simulink model "Tests"  (R2017b)
settings: Solver=FixedStepDiscrete  StartTime=0.0  StopTime=time  FixedStep=0.0025  RelTol=1e-3
InitFcn:
  | time = Data(size(Data,1),1);
values from neighbouring files (symbols this model uses):
  Data = [0 0.0025 0.005 0.0075 0.01 0.0125 0.015 0.0175 0.02 0.0225 0.025 0.0275 ... (231351 elements, 3453x67)]    [apAerobi_0.mat]    (also in apAerobi_3.mat = [0 0.0025 0.005 0.0075 0.01 0.0125 0.015 0.0175 0.02 0.0225 ; apAerobi_4.mat = [0 0.0025 0.005 0.0075 0.01 0.0125 0.015 0.0175 0.02 0.0225 )
libraries: simulink x25
settings Model: Creator=GRVC  LastModifiedBy=root
settings CodeAppCC: StateflowObjectComments=on

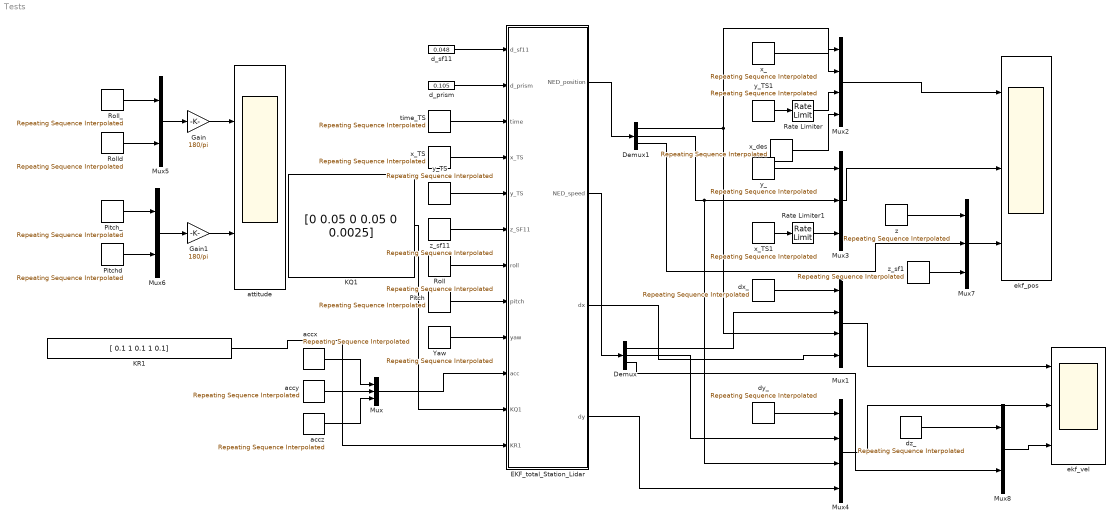
== system Tests ==
  Demux : Demux  Outputs=3
  Demux1 : Demux  Outputs=3
  EKF_total_Station_Lidar : Subsystem
  Gain : Gain  Gain=180/pi
  Gain1 : Gain  Gain=180/pi
  KQ1 : Constant  Value="[0 0.05  0 0.05 0 0.0025]"
  KR1 : Constant  Value=[ 0.1 1 0.1 1 0.1]
  Mux : Mux  Inputs=3
  Mux1 : Mux
  Mux2 : Mux
  Mux3 : Mux  Inputs=3
  Mux4 : Mux
  Mux5 : Mux  Inputs=2
  Mux6 : Mux  Inputs=2
  Mux7 : Mux  Inputs=3
  Mux8 : Mux  Inputs=2
  Pitch : simulink/Sources/Repeating Sequence Interpolated  OutValues=Data(:,3)  TimeValues=Data(:,1)  LookUpMeth=Interpolation-Use End Values  tsamp=0.0025  OutMin=[]  OutMax=[]  OutDataTypeStr=double  OutputDataTypeScalingMode=double  OutDataType=fixdt(0,8)  OutScaling=2^-10
  Pitch_ : simulink/Sources/Repeating Sequence Interpolated  OutValues=Data(:,3)  TimeValues=Data(:,1)  LookUpMeth=Interpolation-Use End Values  tsamp=0.0025  OutMin=[]  OutMax=[]  OutDataTypeStr=double  OutputDataTypeScalingMode=double  OutDataType=fixdt(0,8)  OutScaling=2^-10
  Pitchd : simulink/Sources/Repeating Sequence Interpolated  OutValues=Data(:,49)  TimeValues=Data(:,1)  LookUpMeth=Interpolation-Use End Values  tsamp=0.0025  OutMin=[]  OutMax=[]  OutDataTypeStr=double  OutputDataTypeScalingMode=double  OutDataType=fixdt(0,8)  OutScaling=2^-10
  Rate Limiter : RateLimiter  RisingSlewLimit=10  FallingSlewLimit=-10  SampleTimeMode=inherited
  Rate Limiter1 : RateLimiter  RisingSlewLimit=10  FallingSlewLimit=-10  SampleTimeMode=inherited
  Roll : simulink/Sources/Repeating Sequence Interpolated  OutValues=Data(:,2)  TimeValues=Data(:,1)  LookUpMeth=Interpolation-Use End Values  tsamp=0.0025  OutMin=[]  OutMax=[]  OutDataTypeStr=double  OutputDataTypeScalingMode=double  OutDataType=fixdt(0,8)  OutScaling=2^-10
  Roll_ : simulink/Sources/Repeating Sequence Interpolated  OutValues=Data(:,2)  TimeValues=Data(:,1)  LookUpMeth=Interpolation-Use End Values  tsamp=0.0025  OutMin=[]  OutMax=[]  OutDataTypeStr=double  OutputDataTypeScalingMode=double  OutDataType=fixdt(0,8)  OutScaling=2^-10
  Rolld : simulink/Sources/Repeating Sequence Interpolated  OutValues=Data(:,48)  TimeValues=Data(:,1)  LookUpMeth=Interpolation-Use End Values  tsamp=0.0025  OutMin=[]  OutMax=[]  OutDataTypeStr=double  OutputDataTypeScalingMode=double  OutDataType=fixdt(0,8)  OutScaling=2^-10
  Yaw : simulink/Sources/Repeating Sequence Interpolated  OutValues=Data(:,4)  TimeValues=Data(:,1)  LookUpMeth=Interpolation-Use End Values  tsamp=0.0025  OutMin=[]  OutMax=[]  OutDataTypeStr=double  OutputDataTypeScalingMode=double  OutDataType=fixdt(0,8)  OutScaling=2^-10
  accx : simulink/Sources/Repeating Sequence Interpolated  OutValues=Data(:,8)  TimeValues=Data(:,1)  LookUpMeth=Interpolation-Use End Values  tsamp=0.0025  OutMin=[]  OutMax=[]  OutDataTypeStr=double  OutputDataTypeScalingMode=double  OutDataType=fixdt(0,8)  OutScaling=2^-10
  accy : simulink/Sources/Repeating Sequence Interpolated  OutValues=Data(:,9)  TimeValues=Data(:,1)  LookUpMeth=Interpolation-Use End Values  tsamp=0.0025  OutMin=[]  OutMax=[]  OutDataTypeStr=double  OutputDataTypeScalingMode=double  OutDataType=fixdt(0,8)  OutScaling=2^-10
  accz : simulink/Sources/Repeating Sequence Interpolated  OutValues=Data(:,10)  TimeValues=Data(:,1)  LookUpMeth=Interpolation-Use End Values  tsamp=0.0025  OutMin=[]  OutMax=[]  OutDataTypeStr=double  OutputDataTypeScalingMode=double  OutDataType=fixdt(0,8)  OutScaling=2^-10
  attitude : Scope  NumInputPorts=2
  d_prism : Constant  Value=0.105
  d_sf11 : Constant  Value=0.048
  dx_ : simulink/Sources/Repeating Sequence Interpolated  OutValues=Data(:,33)  TimeValues=Data(:,1)  LookUpMeth=Interpolation-Use End Values  tsamp=0.0025  OutMin=[]  OutMax=[]  OutDataTypeStr=double  OutputDataTypeScalingMode=double  OutDataType=fixdt(0,8)  OutScaling=2^-10
  dy_ : simulink/Sources/Repeating Sequence Interpolated  OutValues=Data(:,34)  TimeValues=Data(:,1)  LookUpMeth=Interpolation-Use End Values  tsamp=0.0025  OutMin=[]  OutMax=[]  OutDataTypeStr=double  OutputDataTypeScalingMode=double  OutDataType=fixdt(0,8)  OutScaling=2^-10
  dz_ : simulink/Sources/Repeating Sequence Interpolated  OutValues=Data(:,35)  TimeValues=Data(:,1)  LookUpMeth=Interpolation-Use End Values  tsamp=0.0025  OutMin=[]  OutMax=[]  OutDataTypeStr=double  OutputDataTypeScalingMode=double  OutDataType=fixdt(0,8)  OutScaling=2^-10
  ekf_pos : Scope  NumInputPorts=3
  ekf_vel : Scope  NumInputPorts=3
  time_TS : simulink/Sources/Repeating Sequence Interpolated  OutValues=Data(:,40)  TimeValues=Data(:,1)  LookUpMeth=Interpolation-Use End Values  tsamp=0.0025  OutMin=[]  OutMax=[]  OutDataTypeStr=double  OutputDataTypeScalingMode=double  OutDataType=fixdt(0,8)  OutScaling=2^-10
  x_ : simulink/Sources/Repeating Sequence Interpolated  OutValues=Data(:,30)  TimeValues=Data(:,1)  LookUpMeth=Interpolation-Use End Values  tsamp=0.0025  OutMin=[]  OutMax=[]  OutDataTypeStr=double  OutputDataTypeScalingMode=double  OutDataType=fixdt(0,8)  OutScaling=2^-10
  x_TS : simulink/Sources/Repeating Sequence Interpolated  OutValues=Data(:,37)  TimeValues=Data(:,1)  LookUpMeth=Interpolation-Use End Values  tsamp=0.0025  OutMin=[]  OutMax=[]  OutDataTypeStr=double  OutputDataTypeScalingMode=double  OutDataType=fixdt(0,8)  OutScaling=2^-10
  x_TS1 : simulink/Sources/Repeating Sequence Interpolated  OutValues=Data(:,37)  TimeValues=Data(:,1)  LookUpMeth=Interpolation-Use End Values  tsamp=0.0025  OutMin=[]  OutMax=[]  OutDataTypeStr=double  OutputDataTypeScalingMode=double  OutDataType=fixdt(0,8)  OutScaling=2^-10
  x_des : simulink/Sources/Repeating Sequence Interpolated  OutValues=Data(:,41)  TimeValues=Data(:,1)  LookUpMeth=Interpolation-Use End Values  tsamp=0.0025  OutMin=[]  OutMax=[]  OutDataTypeStr=double  OutputDataTypeScalingMode=double  OutDataType=fixdt(0,8)  OutScaling=2^-10
  y_ : simulink/Sources/Repeating Sequence Interpolated  OutValues=Data(:,31)  TimeValues=Data(:,1)  LookUpMeth=Interpolation-Use End Values  tsamp=0.0025  OutMin=[]  OutMax=[]  OutDataTypeStr=double  OutputDataTypeScalingMode=double  OutDataType=fixdt(0,8)  OutScaling=2^-10
  y_TS : simulink/Sources/Repeating Sequence Interpolated  OutValues=Data(:,38)  TimeValues=Data(:,1)  LookUpMeth=Interpolation-Use End Values  tsamp=0.0025  OutMin=[]  OutMax=[]  OutDataTypeStr=double  OutputDataTypeScalingMode=double  OutDataType=fixdt(0,8)  OutScaling=2^-10
  y_TS1 : simulink/Sources/Repeating Sequence Interpolated  OutValues=Data(:,38)  TimeValues=Data(:,1)  LookUpMeth=Interpolation-Use End Values  tsamp=0.0025  OutMin=[]  OutMax=[]  OutDataTypeStr=double  OutputDataTypeScalingMode=double  OutDataType=fixdt(0,8)  OutScaling=2^-10
  z : simulink/Sources/Repeating Sequence Interpolated  OutValues=Data(:,32)  TimeValues=Data(:,1)  LookUpMeth=Interpolation-Use End Values  tsamp=0.0025  OutMin=[]  OutMax=[]  OutDataTypeStr=double  OutputDataTypeScalingMode=double  OutDataType=fixdt(0,8)  OutScaling=2^-10
  z_sf1 : simulink/Sources/Repeating Sequence Interpolated  OutValues=Data(:,36)  TimeValues=Data(:,1)  LookUpMeth=Interpolation-Use End Values  tsamp=0.0025  OutMin=[]  OutMax=[]  OutDataTypeStr=double  OutputDataTypeScalingMode=double  OutDataType=fixdt(0,8)  OutScaling=2^-10
  z_sf11 : simulink/Sources/Repeating Sequence Interpolated  OutValues=Data(:,36)  TimeValues=Data(:,1)  LookUpMeth=Interpolation-Use End Values  tsamp=0.0025  OutMin=[]  OutMax=[]  OutDataTypeStr=double  OutputDataTypeScalingMode=double  OutDataType=fixdt(0,8)  OutScaling=2^-10
  wires:
  accy/1 -> Mux/2
  accz/1 -> Mux/3
  accx/1 -> Mux/1
  Mux/1 -> EKF_total_Station_Lidar/10(acc)
  time_TS/1 -> EKF_total_Station_Lidar/3(time)
  d_sf11/1 -> EKF_total_Station_Lidar/1(d_sf11)
  d_prism/1 -> EKF_total_Station_Lidar/2(d_prism)
  z_sf11/1 -> EKF_total_Station_Lidar/6(z_SF11)
  Roll/1 -> EKF_total_Station_Lidar/7(roll)
  Pitch/1 -> EKF_total_Station_Lidar/8(pitch)
  Yaw/1 -> EKF_total_Station_Lidar/9(yaw)
  Mux2/1 -> ekf_pos/1
  Mux3/1 -> ekf_pos/2
  Mux1/1 -> ekf_vel/1
  Mux4/1 -> ekf_vel/2
  dx_/1 -> Mux1/1
  EKF_total_Station_Lidar/1(NED_position) -> Demux1/1
  Demux/1 -> Mux1/2
  Demux/2 -> Mux4/2
  x_/1 -> Mux2/1
  y_/1 -> Mux3/1
  Demux/3 -> Mux8/2
  Demux1/3 -> Mux7/2
  dy_/1 -> Mux4/1
  y_TS1/1 -> Rate Limiter/1
  x_TS1/1 -> Rate Limiter1/1
  Rate Limiter/1 -> Mux2/3
  Rate Limiter1/1 -> Mux3/3
  Rolld/1 -> Mux5/2
  Roll_/1 -> Mux5/1
  Mux5/1 -> Gain/1
  Mux6/1 -> Gain1/1
  Pitchd/1 -> Mux6/2
  Pitch_/1 -> Mux6/1
  Demux1/1 -> Mux1/3, Mux2/2
  Demux1/2 -> Mux4/3, Mux3/2
  y_TS/1 -> EKF_total_Station_Lidar/5(y_TS)
  x_TS/1 -> EKF_total_Station_Lidar/4(x_TS)
  EKF_total_Station_Lidar/2(NED_speed) -> Demux/1
  KR1/1 -> EKF_total_Station_Lidar/12(KR1)
  KQ1/1 -> EKF_total_Station_Lidar/11(KQ1)
  Mux7/1 -> ekf_pos/3
  z_sf1/1 -> Mux7/3
  z/1 -> Mux7/1
  Mux8/1 -> ekf_vel/3
  dz_/1 -> Mux8/1
  Gain/1 -> attitude/1
  Gain1/1 -> attitude/2
  x_des/1 -> Mux2/4
  EKF_total_Station_Lidar/3(dx) -> Mux1/4
  EKF_total_Station_Lidar/4(dy) -> Mux4/4

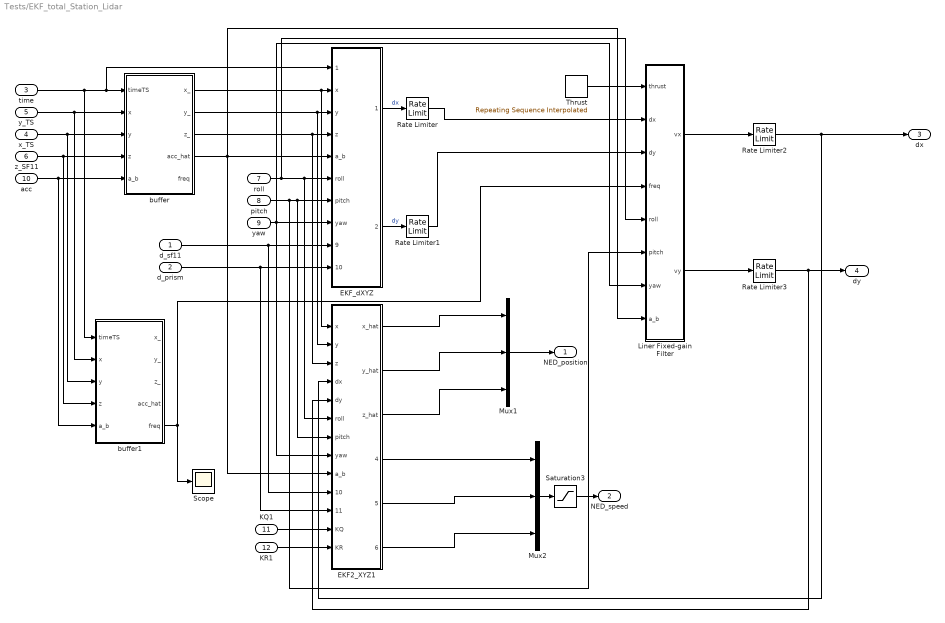
== system Tests/EKF_total_Station_Lidar ==
  d_sf11 : Inport
  d_prism : Inport  Port=2
  time : Inport  Port=3
  x_TS : Inport  Port=4
  y_TS : Inport  Port=5
  z_SF11 : Inport  Port=6
  roll : Inport  Port=7
  pitch : Inport  Port=8
  yaw : Inport  Port=9
  acc : Inport  Port=10
  KQ1 : Inport  Port=11
  KR1 : Inport  Port=12
  EKF2_XYZ1 : MATLAB Function  TreatAsAtomicUnit=on
  EKF_dXYZ : MATLAB Function  TreatAsAtomicUnit=on
  Liner Fixed-gain Filter : MATLAB Function  TreatAsAtomicUnit=on
  Mux1 : Mux  Inputs=3
  Mux2 : Mux  Inputs=3
  Rate Limiter{,1..3} (4 alike) : RateLimiter  RisingSlewLimit=5  FallingSlewLimit=-5  SampleTimeMode=inherited
  Saturation3 : Saturate  UpperLimit=10  LowerLimit=-10
  Scope : Scope
  Thrust : simulink/Sources/Repeating Sequence Interpolated  OutValues=Data(:,45)  TimeValues=Data(:,1)  LookUpMeth=Interpolation-Use End Values  tsamp=0.0025  OutMin=[]  OutMax=[]  OutDataTypeStr=double  OutputDataTypeScalingMode=double  OutDataType=fixdt(0,8)  OutScaling=2^-10
  buffer : MATLAB Function  TreatAsAtomicUnit=on
  buffer1 : MATLAB Function  TreatAsAtomicUnit=on
  NED_position : Outport
  NED_speed : Outport  Port=2
  dx : Outport  Port=3
  dy : Outport  Port=4
  wires:
  Mux1/1 -> NED_position/1
  Mux2/1 -> Saturation3/1
  x_TS/1 -> buffer1/3(y), buffer/3(y)
  y_TS/1 -> buffer/2(x), buffer1/2(x)
  z_SF11/1 -> buffer1/4(z), buffer/4(z)
  acc/1 -> buffer1/5(a_b), buffer/5(a_b)
  buffer/4(acc_hat) -> EKF2_XYZ1/9(a_b), Liner Fixed-gain Filter/8(a_b), EKF_dXYZ/5(a_b)
  EKF_dXYZ/1(dx_hat) -> Rate Limiter/1  "dx"
  EKF_dXYZ/2(dy_hat) -> Rate Limiter1/1  "dy"
  roll/1 -> Liner Fixed-gain Filter/5(roll), EKF2_XYZ1/6(roll), EKF_dXYZ/6(roll)
  pitch/1 -> Liner Fixed-gain Filter/6(pitch), EKF2_XYZ1/7(pitch), EKF_dXYZ/7(pitch)
  yaw/1 -> EKF2_XYZ1/8(yaw), Liner Fixed-gain Filter/7(yaw), EKF_dXYZ/8(yaw)
  d_sf11/1 -> EKF2_XYZ1/10(d_sf11), EKF_dXYZ/9(d_sf11)
  d_prism/1 -> EKF2_XYZ1/11(d_prism), EKF_dXYZ/10(d_prism)
  KQ1/1 -> EKF2_XYZ1/12(KQ)
  KR1/1 -> EKF2_XYZ1/13(KR)
  EKF2_XYZ1/1(x_hat) -> Mux1/1
  EKF2_XYZ1/2(y_hat) -> Mux1/2
  EKF2_XYZ1/3(z_hat) -> Mux1/3
  EKF2_XYZ1/4(dx_hat) -> Mux2/1
  EKF2_XYZ1/5(dy_hat) -> Mux2/2
  EKF2_XYZ1/6(dz_hat) -> Mux2/3
  Saturation3/1 -> NED_speed/1
  time/1 -> buffer1/1(timeTS), EKF_dXYZ/1(timeTS), buffer/1(timeTS)
  buffer/2(y_) -> EKF2_XYZ1/2(y), EKF_dXYZ/3(y)
  buffer/1(x_) -> EKF2_XYZ1/1(x), EKF_dXYZ/2(x)
  buffer/3(z_) -> EKF2_XYZ1/3(z), EKF_dXYZ/4(z)
  Liner Fixed-gain Filter/1(vx) -> Rate Limiter2/1
  Liner Fixed-gain Filter/2(vy) -> Rate Limiter3/1
  Rate Limiter/1 -> Liner Fixed-gain Filter/2(dx)
  Rate Limiter1/1 -> Liner Fixed-gain Filter/3(dy)
  Thrust/1 -> Liner Fixed-gain Filter/1(thrust)
  Rate Limiter2/1 -> EKF2_XYZ1/4(dx), dx/1
  Rate Limiter3/1 -> EKF2_XYZ1/5(dy), dy/1
  buffer1/5(freq) -> Liner Fixed-gain Filter/4(freq), Scope/1

== matlab function Tests/EKF_total_Station_Lidar/EKF_dXYZ ==
  data: timeTS input; x input; y input; z input; a_b input; roll input; pitch input; yaw input; d_sf11 input; d_prism input; dx_hat output; dy_hat output
function [dx_hat,dy_hat] = EKF(timeTS,x,y,z,a_b,roll,pitch,yaw,d_sf11,d_prism)

dt = 0.0025;


a_I = [(a_b(2)-sin(pitch))*cos(yaw)-sin(yaw)*((a_b(1)+sin(roll)*cos(pitch)));
        sin(yaw)*(a_b(2)-sin(pitch))+cos(yaw)*((a_b(1)+sin(roll)*cos(pitch)));
        a_b(3)-cos(roll)*cos(pitch)];

persistent time timeTS0 dx_k dP_k queue_dx queue_dP index Ndata timefreq
if isempty(dx_k) || isempty(dP_k)||isempty(time)|| isempty(timeTS0)|| isempty(queue_dx)|| isempty(queue_dP)|| isempty(index)|| isempty(timefreq)|| isempty(Ndata)

    dx_k = [0;0;0;0;z;0];  
    dP_k = eye(6,6);
    queue_dx = zeros(6,10);
    queue_dP = zeros(6,6,10);

    time = 0;
    timeTS0 = timeTS;
    index = 0;
    timefreq = 0;
    Ndata = 0;

else
    z_corr = d_sf11*sin(roll);
    x_corr = d_prism*cos(yaw);
    y_corr = d_prism*sin(yaw);
    z = (z*cos(roll)+z_corr)*cos(pitch);
    x = x+x_corr;
    y = y+y_corr;
    if timeTS~=0
        if timeTS0~=timeTS
            T = time;
            time = 0;
            timeTS0=timeTS;

            dF = [1 T  0 0  0 0;
                  0 1  0 0  0 0;
                  0 0  1 T  0 0;
                  0 0  0 1  0 0;
                  0 0  0 0  1 T;
                  0 0  0 0  0 1];
            dB = [0.5*T^2       0       0;
                       T       0       0;
                       0  0.5*T^2       0;
                       0        T       0;
                       0        0 0.5*T^2;
                       0        0       T];
            dw_k = [a_I(1);a_I(2);a_I(3)];
            dz_k = [x;y;z];
            dy_k = [dx_k(1);dx_k(3);dx_k(5)];
            dH =[1   0 0  0 0  0;
                0   0 1  0 0  0;
                0   0 0  0 1  0];
            dQ = diag([0 0.05  0 0.05 0 0.05]);
            dR = diag([0.001 0.001 0.001]);
            
        %---------PREDICTION---------%
        %1. Project the state ahead
            dx_k = dF * dx_k + dB * dw_k;
        %2. Project the error covariance ahead
            dP_k = dF * dP_k * dF' + dQ;  
        %--------CORRECTION----------%
        %1. Compute the Kalman Gain
            dK_k = dP_k * dH' / (dH*dP_k*dH' + dR);
            %resid = [sqrt(x0^2+y0^2);atan2(y0,x0);z0] - y_k;
            dresid = dz_k - dy_k;
        %2. Update the estimate via measurement
            dx_k = dx_k +dK_k * dresid;
        %3. Update the error covariance
            dP_k = (eye(size(dK_k,1)) - dK_k * dH) * dP_k;
            
            index = index + 1;

            if index > 10
                queue_dx(:,1) =  dx_k;
                queue_dP(:,:,1) = dP_k;
                index = 1;
            else
                queue_dx(:,index) =  dx_k;
                queue_dP(:,:,index) = dP_k;
            end

        else
            time = time + dt;
        end
   end  

end
dx_hat = dx_k(2);
dy_hat = dx_k(4);

== matlab function Tests/EKF_total_Station_Lidar/buffer1 ==
  data: timeTS input; x_ output; x input; y input; z input; y_ output; z_ output; acc_hat output; freq output; a_b input
function [x_,y_,z_,acc_hat,freq] = data_buffer(timeTS,x,y,z,a_b)

dt = 0.0025;
persistent buffer time index counter t0 total acc_
if isempty(buffer)||isempty(time)||isempty(index)||isempty(counter)||isempty(t0)||isempty(total)||isempty(acc_)
    buffer = zeros(3,20);
    
    time = 0;
    index = 1;
    counter = zeros(1,20);
    if timeTS ~= 0
        buffer(:,index) = [x;y;z];
        counter(1) = 1;
    end
    total = 0;
    t0 = timeTS;
   
    acc_ = [0;0;1];
        
else
    alpha = 0.2;
    a_b = a_b/norm(a_b);
    acc_ = (a_b * alpha) + (acc_ * (1.0 - alpha));
    time = time + dt;
    if time > 0.05
        time = 0;
        if (buffer(1,index) ~= x || buffer(2,index) ~= y )
            buffer(:,index) = [x;y;z];
            counter(index) = 1;
        else

            buffer(:,index) = [x;y;z];
            counter(index) = 0;
        end
        if index == 20
            index = 1;
        else
            index = index + 1;
        end

    end
 
    
end
    freq =sum(counter);
    if freq > 20
        freq = 20;
    end
    if isnan(x) || isnan(y) || isinf(x) || isinf(y) || abs(x) > 50 || abs(y) > 50
        if index <= 1
            x_ = buffer(1,10);
            y_ = buffer(2,10);
        else       
            x_ = buffer(1,index-1);
            y_ = buffer(2,index-1);
        end
        z_ = z;
    else
        if z < 0.3
            z_ = 0.3;
        else
            z_ = z;
        end
        x_ = x;
        y_ = y;   
    end
    acc_hat = acc_;
end

== matlab function Tests/EKF_total_Station_Lidar/buffer ==
  data: timeTS input; x_ output; x input; y input; z input; y_ output; z_ output; acc_hat output; freq output; a_b input
function [x_,y_,z_,acc_hat,freq] = data_buffer(timeTS,x,y,z,a_b)

dt = 0.0025;
persistent buffer time index counter t0 total acc_
if isempty(buffer)||isempty(time)||isempty(index)||isempty(counter)||isempty(t0)||isempty(total)||isempty(acc_)
    buffer = zeros(3,20);
    time = 0;
    index = 1;
    counter = 0;
    if timeTS ~= 0
        buffer(:,index) = [x;y;z];
        counter = 1;
    end
    total = counter;
    t0 = timeTS;
   
    acc_ = [0;0;1];
        
else
    alpha = 0.2;
    a_b = a_b/norm(a_b);
    acc_ = (a_b * alpha) + (acc_ * (1.0 - alpha));
    time = time + dt;
    if timeTS ~= 0 && timeTS <= 1e13        
        if time > 0.5
            %counter = index - 1;
            total = counter;
            counter = 0;
            time = 0;                  
            index = 0;
        else
            
            if index == 0
                if (buffer(1,10) ~= x || buffer(2,10) ~= y )
                    counter = counter+1;
                    buffer(:,1) = [x;y;z];
                    index = 1;
                end
            elseif index >= 10  
                if (buffer(1,10) ~= x || buffer(2,10) ~= y )
                    counter = counter+1;
                    buffer(:,1) = [x;y;z];
                    index = 1;
                end
            else
                if (buffer(1,index) ~= x || buffer(2,index) ~= y )
                    index = index + 1;
                    counter = counter+1;                   
                    buffer(:,index) = [x;y;z];                    
                end
            end
        end

    elseif timeTS == 0
        if time > 0.5
            time = 0;
            index = 0;
            total = counter;
            counter = 0;
        end
    else
        if time > 0.5
            %counter = index - 1;
            total = counter;
            counter = 0;
            time = 0;
            index = 0;
        end
        
    end

    
end
    freq =total/0.5;
    if freq > 20
        freq = 20;
    end
    if isnan(x) || isnan(y) || isinf(x) || isinf(y) || abs(x) > 50 || abs(y) > 50
        if index <= 1
            x_ = buffer(1,10);
            y_ = buffer(2,10);
        else       
            x_ = buffer(1,index-1);
            y_ = buffer(2,index-1);
        end
        z_ = z;
    else
        if z < 0.3
            z_ = 0.3;
        else
            z_ = z;
        end
        x_ = x;
        y_ = y;   
    end
    acc_hat = acc_;
end

== matlab function Tests/EKF_total_Station_Lidar/Liner Fixed-gain Filter ==
  data: thrust input; dx input; dy input; freq input; roll input; pitch input; yaw input; a_b input; vx output; vy output
function [vx,vy] = linear_Fixed_Gain_Filter(thrust,dx,dy,freq,roll,pitch,yaw,a_b)

dt = 0.0025;
m = 2.5;
mu = 0.87;
R_yaw = [cos(yaw) -sin(yaw);sin(yaw) cos(yaw)];  
persistent x_k P_k
if isempty(x_k)||isempty(P_k)
    x_k = [0;0];
    P_k = [1 0;0 1;];
        
else
    if thrust < 40
        thrust = 40;
    elseif thrust >120
        thrust = 120;
    end
    u = 62.5/thrust;
    
    
    a_I = [a_b(2)-sin(pitch);
           a_b(1)+sin(roll)*cos(pitch);
           a_b(3)-cos(roll)*cos(pitch)];

      
    x_I = R_yaw*[dx;dy];
    
    F = [(mu*u)/m          0;
                0   (mu*u)/m];
    
    H = [(mu*u)/m          0; 
                0   (mu*u)/m; 
                dt          0;
                0          dt;];
            
    Q = diag([1 1]);
    if freq >= 20
        R = diag([0.5 0.5 0.004 0.004]);
    else
        R = diag([0.01 0.01 100000 100000]);
    end
    
    z_k = [a_I(1);a_I(2);x_I(1);x_I(2)];
    y_k = x_k;
        %---------PREDICTION---------%
    %1. Project the state ahead
        x_k = F * x_k;% + B * w_k;
    %2. Project the error covariance ahead
        P_k = F * P_k * F' + Q;  
    %--------CORRECTION----------%
    %1. Compute the Kalman Gain
        K_k = P_k * H' / (H*P_k*H' + R);
        
        resid = z_k - H*y_k;
    %2. Update the estimate via measurement
        x_k = x_k + K_k * resid;
    %3. Update the error covariance
        P_k = (eye(size(K_k,1)) - K_k * H) * P_k;    
    
 
end
v = R_yaw'*x_k;
vx = v(1);
vy = v(2);

== matlab function Tests/EKF_total_Station_Lidar/EKF2_XYZ1 ==
  data: x_hat output; y_hat output; z_hat output; x input; y input; z input; dx input; dy input; roll input; pitch input; yaw input; a_b input; d_sf11 input; d_prism input; KQ input; KR input; dx_hat output; dy_hat output; dz_hat output
function [x_hat,y_hat,z_hat,dx_hat,dy_hat,dz_hat] = EKF(x,y,z,dx,dy,roll,pitch,yaw,a_b,d_sf11,d_prism,KQ,KR)

dt = 0.0025;

a_I = [(a_b(2)-sin(pitch))*cos(yaw)-sin(yaw)*((a_b(1)+sin(roll)*cos(pitch)));
        sin(yaw)*(a_b(2)-sin(pitch))+cos(yaw)*((a_b(1)+sin(roll)*cos(pitch)));
        a_b(3)-cos(roll)*cos(pitch)];

persistent  x_k P_k x0 y0 z0 
if isempty(x_k) || isempty(P_k)|| isempty(x0)|| isempty(y0)|| isempty(z0)
    x_k = [0;0;0;0;z;0];  
    P_k = eye(6,6);
    x0 = 0;
    y0 = 0;
    z0 = 0;
else
    z_corr = d_sf11*sin(roll);
    x_corr = d_prism*cos(yaw);
    y_corr = d_prism*sin(yaw);
    z0 = (z*cos(roll)+z_corr)*cos(pitch);
    x0 = x+x_corr;
    y0 = y+y_corr;
        F = [1 dt 0  0 0 0;
             0  1 0  0 0 0;
             0  0 1 dt 0 0;
             0  0 0  1 0 0;
             0  0 0  0 1 dt;
             0  0 0  0 0 1];
        B = [0.5*dt^2       0       0;
                   dt       0       0;
                   0 0.5*dt^2       0;
                   0       dt       0;
                   0       0 0.5*dt^2;
                   0       0       dt];
        w_k = [a_I(1);a_I(2);a_I(3)];        
        z_k = [x0;dx;y0;dy;z0;];
        y_k = [x_k(1);x_k(2);x_k(3);x_k(4);x_k(5);];
        H =[1   0 0  0 0  0;
            0   1 0  0 0  0;
            0   0 1  0 0  0;
            0   0 0  1 0  0;
            0   0 0  0 1  0;
            ];
        Q = diag(KQ);
        R = diag(KR);
    %---------PREDICTION---------%
    %1. Project the state ahead
        x_k = F * x_k + B * w_k;
    %2. Project the error covariance ahead
        P_k = F * P_k * F' + Q;  
    %--------CORRECTION----------%
    %1. Compute the Kalman Gain
        K_k = P_k * H' / (H*P_k*H' + R);
        
        resid = z_k - y_k;
    %2. Update the estimate via measurement
        x_k = x_k + K_k * resid;
    %3. Update the error covariance
        P_k = (eye(size(K_k,1)) - K_k * H) * P_k;    

end
x_hat = x_k(1);
y_hat = x_k(3);
z_hat = x_k(5);
dx_hat = x_k(2);
dy_hat = x_k(4);
dz_hat = x_k(6);
